simulink model "MAIN (2)"  (R2023a)
settings: Solver=VariableStepAuto  StartTime=0.0  StopTime=5  RelTol=1e-3
libraries: dspstat3 x4, simulink x2, commchan3 x2, dspvision x2, commblkcod2 x2, commdigbbndpm3 x2, commfilt2 x2, dspquant2 x2, commsink2 x1, commutil2 x1
settings Model: Creator=241pr  LastModifiedBy=241pr

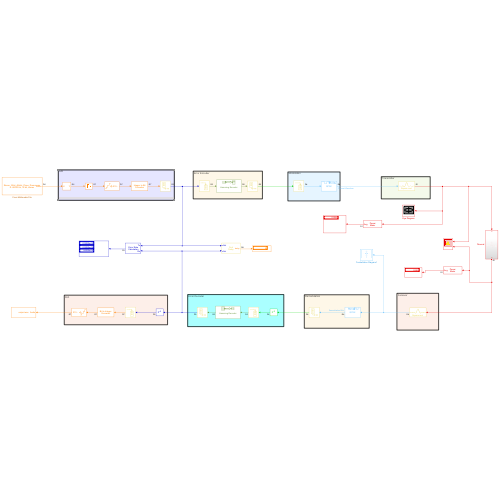
[thumbnail: Simulink's stored preview of the top-level diagram]
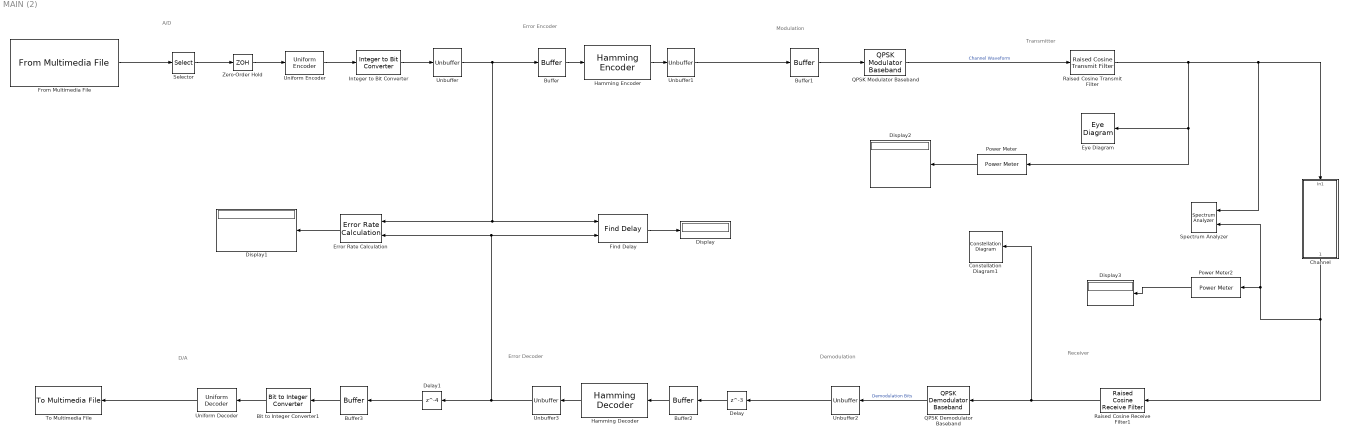
== system MAIN (2) ==
  note: Receiver
  note: Transmitter
  note: Demodulation
  note: Error Encoder
  note: A/D
  note: Error Decoder
  note: Modulation
  note: D/A
  Bit to Integer Converter1 : simulink/Logic and Bit Operations/Bit to Integer Converter  nbits=8  bitOrder=MSB first  signedOutputValues=Signed  outDtype=Inherit via internal rule  outDtypeSigned=int32
  Buffer : Buffer  N=4  OutputFrames=off
  Buffer1 : Buffer  N=2  OutputFrames=off
  Buffer2 : Buffer  N=7  OutputFrames=off
  Buffer3 : Buffer  N=8  OutputFrames=off
  Channel : Subsystem
  Constellation Diagram1 : ConstellationDiagram  WindowPosition=[1.000000,41.000000,1920.000000,1017.000000,]  Visible=on  ScopeFrameLocation=window  SamplesPerSymbol=4  SymbolsToDisplaySource=Property  SymbolsToDisplay=100000  ReferenceConstellation=QPSK  XLimits=[-3.53,3.53]  YLimits=[-5.16,5.17]  ShowLegend=on  EnableMeasurements=on  DefaultConfigurationName=comm.scopes.ConstellationDiagramBlockCfg
  Delay : Delay  DelayLength=3
  Delay1 : Delay  DelayLength=4
  Display{,1..3} (4 alike) : Display
      Display1 settings: Format=short_e
  Error Rate Calculation : commsink2/Error Rate Calculation  N=20  st_delay=0  cp_mode=Entire frame  subframe=[]  PMode=Port  WsName=ErrorVec  RsMode2=off  stop=off  numErr=100  maxBits=1e6
      settings: LibrarySourceBlock=|
      | commhdlsink/Error Rate
      | Calculation
  Eye Diagram : EyeDiagram
  Find Delay : commutil2/Find Delay  corrLength=200  chgSigOP=off  stopUpdate=off  numConstDelay=3
  From Multimedia File : dspvision/From Multimedia File  inputFilename=C:\Users\241pr\OneDrive - UBC\Desktop\Apps\UBC\ELEC 391\Project\SOUND\Stereo_32bit_48kHz_Piano_Drums.wav  readRange=[1 Inf]  loop=on  numPlays=inf  outputStreams=Audio only  videoDataType=single  audioDataType=double  inheritSampleTime=on  userDefinedSampleTime=1/40  noAudioOutput=off  isIntensityVideo=off  fourcc=RGB  colorVideoFormat=Separate color signals  outputEOF=off  dataOrg=Column-major  audioFrameSize=1  computeAudioFrameSize=off  outSamplingMode=Sample based
  Hamming Decoder : commblkcod2/Hamming Decoder  n=7  k=4
  Hamming Encoder : commblkcod2/Hamming Encoder  n=7  k=4
  Integer to Bit Converter : simulink/Logic and Bit Operations/Integer to Bit Converter  nbits=8  signedInputValues=Signed  bitOrder=MSB first  outDtype=double
  Power Meter : dspstat3/Power Meter  Measurement=Average power  ReferenceLoad=1  OutputPowerUnits=Watts  WindowLength=256  OverlapLength=255  AllowArbitraryInputLength=off  ComputeCCDF=off  PowerRange=50  PowerResolution=0.1  CCDFOutput=Relative power (dB above average power)  ProbabilityVector=[ 10; 1; 0.1; 0.01; 0.001; 0.0001 ]  RelativePowerVector=[ 0; 3; 6; 9; 12 ]  ResetPort=off  SimulateUsing=Code generation
  Power Meter2 : dspstat3/Power Meter  Measurement=Average power  ReferenceLoad=1  OutputPowerUnits=Watts  WindowLength=256  OverlapLength=255  AllowArbitraryInputLength=off  ComputeCCDF=off  PowerRange=50  PowerResolution=0.1  CCDFOutput=Relative power (dB above average power)  ProbabilityVector=[ 10; 1; 0.1; 0.01; 0.001; 0.0001 ]  RelativePowerVector=[ 0; 3; 6; 9; 12 ]  ResetPort=off  SimulateUsing=Code generation
  QPSK Demodulator Baseband : commdigbbndpm3/QPSK Demodulator Baseband  OutType=Bit  DecType=Hard decision  VarSource=Dialog  Variance=1  Dec=Gray  Ph=pi/4  outDtype1=Inherit via internal rule  outDtype2=Inherit via internal rule  derotateFactorWordLen=16  derotateFactorDataTypeStr=Inherit: Same word length as input  derotateFactorLastDataTypeStr=Inherit: Same word length as input
  QPSK Modulator Baseband : commdigbbndpm3/QPSK Modulator Baseband  InType=Bit  Enc=Gray  Ph=pi/4  outDtype=double  outWordLen=16  outUDDataType=sfix(16)  outFracLenMode=Best precision  outFracLen=15  outDataTypeStr=double  outLastDataTypeStr=double
  Raised Cosine Receive Filter1 : commfilt2/Raised Cosine Receive Filter  filtType=Square root  R=0.4  filtSpan=8  N=4  downFactor=4  downOffset=0  filterGain=2  InputProcessing=Columns as channels (frame based)  RateOptions=Allow multirate processing  framing=Mute  checkCoeff=off  variableName=rcRxFilt1  currentFiltSpan=10  D=5  inputOffset=0  sampMode=Mute  saveAsFlag=0  rateMode=Downsampling  checkGain=Normalized  launchFVT=on  roundingMode=Floor  overflowMode=off  coeffDataTypeStr=Inherit: Same word length as input  coeffMin=[]  coeffMax=[]  coeffLastDataTypeStr=Inherit: Same word length as input  accumDataTypeStr=Inherit: Same as product output  accumLastDataTypeStr=Inherit: Same as product output  outputDataTypeStr=Inherit: Same as accumulator  outputMin=[]  outputMax=[]  outputLastDataTypeStr=Inherit: Same as accumulator
  Raised Cosine Transmit Filter : commfilt2/Raised Cosine Transmit Filter  filtType=Square root  R=0.4  filtSpan=8  N=4  filterGain=2  InputProcessing=Columns as channels (frame based)  RateOptions=Allow multirate processing  framing=Mute  checkCoeff=off  variableName=rcTxFilt  checkGain=Normalized  sampMode=Mute  saveAsFlag=0  currentFiltSpan=10  D=5  launchFVT=on  roundingMode=Floor  overflowMode=off  coeffDataTypeStr=Inherit: Same word length as input  coeffMin=[]  coeffMax=[]  coeffLastDataTypeStr=Inherit: Same word length as input  outputDataTypeStr=Inherit: Same as accumulator  outputMin=[]  outputMax=[]  outputLastDataTypeStr=Inherit: Same as accumulator
  Selector : Selector  NumberOfDimensions=2  IndexMode=Zero-based  InputPortWidth=3  IndexOptions=Select all,Index vector (dialog)  Indices=[1 3],0  OutputSizes=1,1
  Spectrum Analyzer : SpectrumAnalyzer  NumInputPorts=2  WindowPosition=[1.000000,41.000000,1920.000000,1017.000000,]  Visible=on  ScopeFrameLocation=window  SampleRateSource=Property  SampleRate=1200000  AxesScaling=Manual  FrequencySpan=Start and stop frequencies  StartFrequency=0  StopFrequency=600000  AveragingMethod=Exponential  YLimits=[-117.14660311,28.97147385]  ShowLegend=on
  To Multimedia File : dspvision/To Multimedia File  outputFilename=C:\Users\241pr\OneDrive - UBC\Desktop\Apps\UBC\ELEC 391\Project\output.wav  streamSelection=Audio only  videoCompressor=None (uncompressed)  audioCompressor=None (uncompressed)  imagePorts=Separate color signals  fileType=WAV  audioDatatype=8-bit integer  fourcc=RGB  videoQuality=75  mj2000CompFactor=10
  Unbuffer{,1..3} (4 alike) : Unbuffer
  Uniform Decoder : dspquant2/Uniform Decoder  peak=1  bits=8  overflowMode=Wrap  otype=Double
  Uniform Encoder : dspquant2/Uniform Encoder  peak=1  bits=8  otype=Signed integer
  Zero-Order Hold : ZeroOrderHold  SampleTime=1/40000
  wires:
  Error Rate Calculation/1 -> Display1/1
  Unbuffer2/1 -> Delay/1
  Channel/1(1) -> Power Meter2/1, Spectrum Analyzer/2, Raised Cosine Receive Filter1/1
  Find Delay/1 -> Display/1
  Integer to Bit Converter/1 -> Unbuffer/1
  Buffer3/1 -> Bit to Integer Converter1/1
  From Multimedia File/1 -> Selector/1
  Uniform Decoder/1 -> To Multimedia File/1
  Hamming Decoder/1 -> Unbuffer3/1
  Buffer2/1 -> Hamming Decoder/1
  Delay1/1 -> Buffer3/1
  Unbuffer3/1 -> Delay1/1, Error Rate Calculation/2, Find Delay/2
  Unbuffer1/1 -> Buffer1/1
  QPSK Modulator Baseband/1 -> Raised Cosine Transmit Filter/1  "Channel Waveform"
  Bit to Integer Converter1/1 -> Uniform Decoder/1
  Buffer1/1 -> QPSK Modulator Baseband/1
  Uniform Encoder/1 -> Integer to Bit Converter/1
  Delay/1 -> Buffer2/1
  Buffer/1 -> Hamming Encoder/1
  Hamming Encoder/1 -> Unbuffer1/1
  Raised Cosine Transmit Filter/1 -> Eye Diagram/1, Power Meter/1, Spectrum Analyzer/1, Channel/1(In1)
  Zero-Order Hold/1 -> Uniform Encoder/1
  Selector/1 -> Zero-Order Hold/1
  QPSK Demodulator Baseband/1 -> Unbuffer2/1  "Demodulation Bits"
  Raised Cosine Receive Filter1/1 -> Constellation Diagram1/1, QPSK Demodulator Baseband/1
  Unbuffer/1 -> Find Delay/1, Error Rate Calculation/1, Buffer/1
  Power Meter/1 -> Display2/1
  Power Meter2/1 -> Display3/1

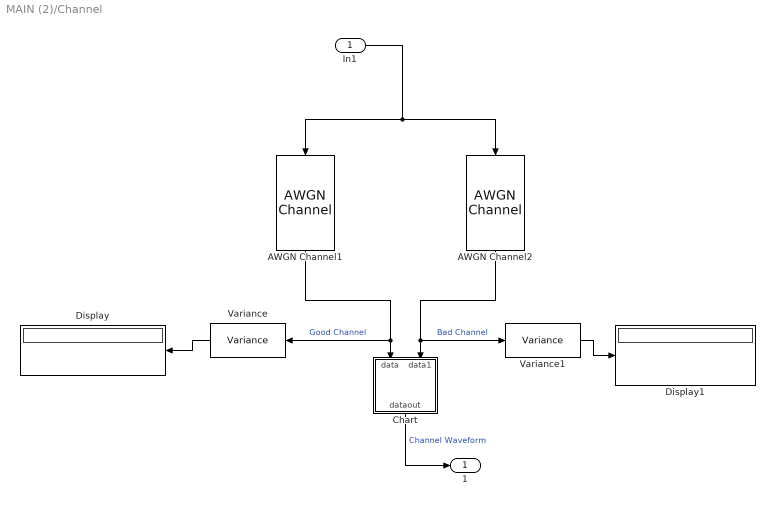
== system MAIN (2)/Channel ==
  In1 : Inport
  AWGN Channel1 : commchan3/AWGN Channel  LegacyMode=on  NoiseMethod="Signal to noise ratio  (SNR)"  noiseMode="Signal to noise ratio  (SNR)"  EbNo=0  EsNo=6  SNR=21  BitsPerSymbol=1  SignalPower=1  SamplesPerSymbol=1  SymbolPeriod=1  VarianceSource=Parameter  Variance=1  RandomStream=Global stream  Seed=67  SimulateUsing=Code generation
  AWGN Channel2 : commchan3/AWGN Channel  LegacyMode=on  NoiseMethod="Signal to noise ratio  (SNR)"  noiseMode="Signal to noise ratio  (SNR)"  EbNo=10  EsNo=10  SNR=9  BitsPerSymbol=1  SignalPower=1  SamplesPerSymbol=1  SymbolPeriod=1  VarianceSource=Parameter  Variance=1  RandomStream=Global stream  Seed=67  SimulateUsing=Code generation
  Chart : Stateflow chart  TreatAsAtomicUnit=on
      settings: PortSchema="{\"entries\":[{\"content\":{\"sides\":[{\"content\":{},\"type\":\"ConnectorPlacement.EquallySpacedRectSide\",\"uuid\":\"e2cc2d5e-5563-4536-8d35-b8bc41da3939\"},{\"content\":{\"side\":\"RIGHT\"},\"type\":\"ConnectorPlacement.EquallySpacedRectSide\",\"uuid\":\"21ece9a8-9882-4ba2-9e27-ace723075a7b\"},{\"content\":{\"connectorIds\":[\"In1\",\"In2\"],\"side\":\"TOP\"},\"type\":\"ConnectorPlacement.EquallySpacedRectSide\",\"uuid\":\"2f00bec1-0aa7-4b8f-8687-0ec56318bf4e\"},{\"content\":{\"connectorIds\":[\"Out1\"],\"side\":\"BOTTOM\"},\"type\":\"ConnectorPlacement.EquallySpacedRectSide\",\"uuid\":\"bac7bfac-b9ec-450e-9076-ded9eacfed37\"}]},\"type\":\"ConnectorPlacement.EquallySpacedConnector\",\"uuid\":\"b35351af-4e23-4d55-8655-919b92b12485\"}],\"packageUris\":[\"http://schema.mathworks.com/mf0/Connector/R2020b\"],\"version\":\"1.0\"}"
  Display : Display
  Display1 : Display
  Variance : dspstat3/Variance  run=off  InputProcessing=Columns as channels (frame based)  reset_popup=None  directionMode=Each column  dimension=1  roiEnable=off  roiType=Rectangles  roiPortion=Entire ROI  roiOutput=Individual statistics for each ROI  roiFlag=off  roundingMode=Floor  overflowMode=off
  Variance1 : dspstat3/Variance  run=off  InputProcessing=Columns as channels (frame based)  reset_popup=None  directionMode=Each column  dimension=1  roiEnable=off  roiType=Rectangles  roiPortion=Entire ROI  roiOutput=Individual statistics for each ROI  roiFlag=off  roundingMode=Floor  overflowMode=off
  1 : Outport
  wires:
  AWGN Channel2/1 -> Variance1/1, Chart/2(data1)  "Bad Channel"
  AWGN Channel1/1 -> Variance/1, Chart/1(data)  "Good Channel"
  Chart/1(dataout) -> 1/1  "Channel Waveform"
  In1/1 -> AWGN Channel1/1, AWGN Channel2/1
  Variance/1 -> Display/1
  Variance1/1 -> Display1/1

== stateflow chart MAIN (2)/Channel/Chart ==
  state Good_Channel
    entry,during:dataout=data
  state Bad_Channel
    entry,during:dataout=data1
  (default) -> Good_Channel : []
  Good_Channel -> Good_Channel [order 2] : after(100,usec)[rand()>0.02]
  Bad_Channel -> Bad_Channel [order 2] : after(100,usec)[rand()>0.24]
  Good_Channel -> Bad_Channel [order 1] : after(100,usec)[rand()<=0.02]
  Bad_Channel -> Good_Channel [order 1] : after(100,usec)[rand()<=0.24]
  data: data input; data1 input; dataout output
